simulink model "SPC_model"  (R2023a)
settings: Solver=VariableStepAuto  StartTime=0.0  StopTime=1000  RelTol=1e-3
values from neighbouring files (symbols this model uses):
  slope = 0    [run_model.m]
libraries: simulink x2, autolibshared x2
settings Model: Creator=jonathan  LastModifiedBy=jonathan
settings SolverCC: ZeroCrossAlgorithm=Adaptive
settings OptimizationCC: ReuseModelBlockBuffer=off
settings DebuggingCC: IgnoredZcDiagnostic=none

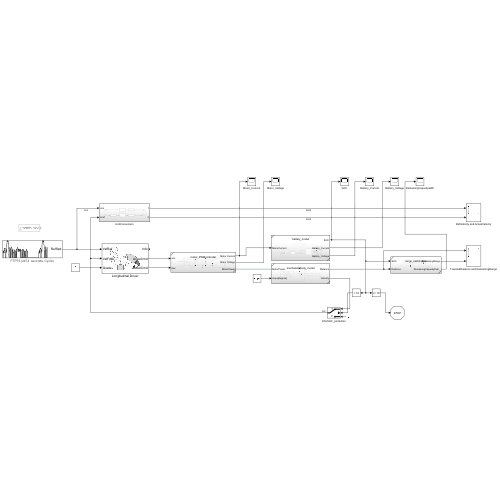
[thumbnail: Simulink's stored preview of the top-level diagram]
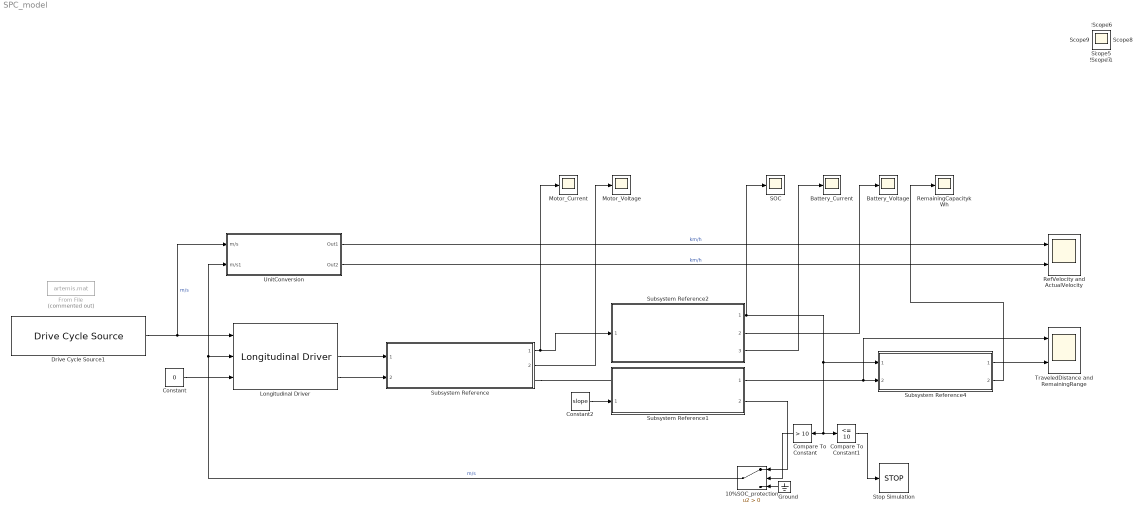
== system SPC_model ==
  10%SOC_protection : Switch  Criteria=u2 > Threshold  SaturateOnIntegerOverflow=off  InputSameDT=off
  Battery_Current : Scope
  Battery_Voltage : Scope
  Compare To Constant : simulink/Logic and Bit Operations/Compare To Constant  relop=>  const=10  OutDataTypeStr=boolean
  Compare To Constant1 : simulink/Logic and Bit Operations/Compare To Constant  relop=<=  const=10  OutDataTypeStr=boolean
  Constant : Constant  Value=0
  Constant2 : Constant  Value=slope
  Drive Cycle Source1 : autolibshared/Drive Cycle Source  cycleVar=FTP75  fileVar=cycleFTP75.mat  tfinal="2474  seconds, Cyclic"  cycleRepeat=on  outAccPort=off  outGearPort=off  gearList=No gear data  t_wot1=5  xdot_woto=0  xdot_wot1=30  t_wot2=20  xdot_wot2=0  t_wotend=30  srcUnit=m/s  outUnit=m/s  srcAccUnit=m/s/s  outAccUnit=m/s^2  dt=0  aMode=2  faultOption=off  velBnd=2  velBndUnit=mph  inUnit=m/s  timeBnd=1  failOption=off  stopSim=off  maxFaultCnt=10  maxFaultTime=2  maxTotFaultTime=15  traceOption=off  dtTrace=1  traceWindow=10  lastDCname=FTP75  lastOutUnit=mph  lastDT=0  lastTB=1  lastSB=2  forceCalcBound=off
      settings: LibrarySourceBlock=vdynlib/Vehicle Scenarios/Drive Cycle and Maneuvers/Drive Cycle Source
  From File : FromFile  Commented=on  FileName=artemis.mat  SampleTime=1  ExtrapolationBeforeFirstDataPoint=Hold first value  ExtrapolationAfterLastDataPoint=Hold last value
  Ground : Ground
  Longitudinal Driver : autolibshared/Longitudinal Driver  extAccelOvr=off  extDecelOvr=off  extAccelHld=off  extDecelHld=off  extAccelZero=off  extDecelZero=off  cntrlType=PI  shftType=None  velUnits=m/s  gearOut=off  Kp=10  Ki=5  Kff=0.1  Kg=0  VehVelVec=[0 100]  KffVec=[.1 .1]  KpVec=[10 10]  KiVec=[5 5]  KgVec=[0 0]  m=1500  Kpt=3000  tau=.1  L=2  aR=200  bR=2.5  cR=.5  g=9.81  vnom=5  Kaw=1  tauerr=.01  tauPt=2  GearInit=0  tShift=.1  pdlVec=[0.1 0.4 0.5 0.9]  upShftTbl=[-1 12.9375 26.4375 39.9375 51.18749999999999 62.4375 72.84375 83.25;-1 16.3125 29.8125 43.3125 54.5624 65.8125 76.78125 87.75;-1 19.6875 33.1875 46.68749999999999 57.9375 69.1875 80.71875 92.25;-1 33 52.5 77.25 100.5 138.75 161.875 185]  dwnShftTbl=[1 9.5625 23.0625 36.5625 47.8125 59.0625 68.90625 78.75;1 12.9375 26.4375 39.9375 51.18749999999999 62.4375 72.84375 83.25;1 16.3125 29.8125 43.3125 54.562499 65.8125 76.78125 87.75;1 19.6875 33.1875 46.68749999999999 57.9375 69.1875 80.71875 92.25]  tClutch=.5  tRev=.5  tPark=120  aMode=2  UpGearVec="[0  1  2  3  4  5  6  7]"  DownGearVec="[1  2  3  4  5  6  7  8]"
      settings: LibrarySourceBlock=vehdynlibdriver/Longitudinal Driver
  Motor_Current : Scope
  Motor_Voltage : Scope
  RefVelocity and ActualVelocity : Scope  NumInputPorts=2
  RemainingCapacitykWh : Scope
  SOC : Scope
  Stop Simulation : Stop
  Subsystem Reference : Subsystem  ReferencedSubsystem=motor_PWMcontroller
  Subsystem Reference1 : Subsystem  ReferencedSubsystem=mechanicalbody_model
      settings: PortSchema="{\"entries\":[{\"content\":{\"sides\":[{\"content\":{\"connectorIds\":[\"LConn1\",\"In1\"]},\"type\":\"ConnectorPlacement.EquallySpacedRectSide\",\"uuid\":\"900da1ad-8a01-4010-b1c0-b1da36539f58\"},{\"content\":{\"connectorIds\":[\"Out1\",\"Out2\"],\"side\":\"RIGHT\"},\"type\":\"ConnectorPlacement.EquallySpacedRectSide\",\"uuid\":\"71df76a2-1493-4f23-928b-eae60623c8a5\"},{\"content\":{\"side\":\"TOP\"},\"type\":\"ConnectorPlacement.EquallySpacedRectSide\",\"uuid\":\"a5e86f98-2844-4158-89f5-dccf43deca94\"}]},\"type\":\"ConnectorPlacement.EquallySpacedConnector\",\"uuid\":\"b0cc335e-0ca0-48bf-99c0-8609726a12ec\"}],\"packageUris\":[\"http://schema.mathworks.com/mf0/Connector/R2020b\"],\"version\":\"1.0\"}"
  Subsystem Reference2 : Subsystem  ReferencedSubsystem=battery_model
  Subsystem Reference4 : Subsystem  ReferencedSubsystem=range_esstimation
  TraveledDistance and RemainingRange : Scope  NumInputPorts=2
  UnitConversion : Subsystem
  Scope{,1..3,5..9,11} (10 alike) : Scope
  wires:
  Constant2/1 -> Subsystem Reference1/1
  Subsystem Reference/1 -> Motor_Current/1, Subsystem Reference2/1
  Ground/1 -> 10%SOC_protection/3
  Compare To Constant/1 -> 10%SOC_protection/2
  Compare To Constant1/1 -> Stop Simulation/1
  Subsystem Reference1/1 -> TraveledDistance and RemainingRange/1, Subsystem Reference4/2
  Longitudinal Driver/2 -> Subsystem Reference/1
  Longitudinal Driver/3 -> Subsystem Reference/2
  Constant/1 -> Longitudinal Driver/3
  Subsystem Reference1/2 -> 10%SOC_protection/1
  Subsystem Reference2/1 -> SOC/1, Compare To Constant1/1, Compare To Constant/1, Subsystem Reference4/1
  Subsystem Reference4/1 -> TraveledDistance and RemainingRange/2
  Drive Cycle Source1/1 -> UnitConversion/1(m/s), Longitudinal Driver/1  "m/s"
  10%SOC_protection/1 -> UnitConversion/2(m/s1), Longitudinal Driver/2  "m/s"
  UnitConversion/1(Out1) -> RefVelocity and ActualVelocity/1  "km/h"
  UnitConversion/2(Out2) -> RefVelocity and ActualVelocity/2  "km/h"
  Subsystem Reference2/2 -> Battery_Voltage/1
  Subsystem Reference2/3 -> Battery_Current/1
  Subsystem Reference/2 -> Motor_Voltage/1
  Subsystem Reference4/2 -> RemainingCapacitykWh/1
  connections:
  Subsystem Reference/RConn1 -- Subsystem Reference1/LConn1

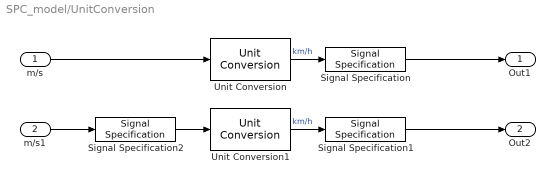
== system SPC_model/UnitConversion ==
  m/s : Inport
  m/s1 : Inport  Port=2
  Signal Specification : SignalSpecification  Unit=km/hr
  Signal Specification1 : SignalSpecification  Unit=km/hr
  Signal Specification2 : SignalSpecification  Unit=m/s
  Unit Conversion : UnitConversion  OutputType=Inherit: Inherit via back propagation
  Unit Conversion1 : UnitConversion  OutputType=Inherit: Inherit via back propagation
  Out1 : Outport
  Out2 : Outport  Port=2
  wires:
  Signal Specification2/1 -> Unit Conversion1/1
  Unit Conversion/1 -> Signal Specification/1  "km/h"
  Signal Specification1/1 -> Out2/1
  Unit Conversion1/1 -> Signal Specification1/1  "km/h"
  m/s/1 -> Unit Conversion/1
  m/s1/1 -> Signal Specification2/1
  Signal Specification/1 -> Out1/1
